simulink model "OFDM_256_pilots"  (R2018b)
settings: Solver=VariableStepAuto  StartTime=0.0  StopTime=inf  RelTol=1e-3
PreLoadFcn:
  | M=16;
  | Fs=1e7;
undefined symbols (not defined in the file): EbNo
libraries: commutil2 x2, commsink2 x2, commofdm x2, commdigbbndam3 x2, commchan3 x1, commrandsrc3 x1
settings Model: Creator=HOBA  LastModifiedBy=HOBA

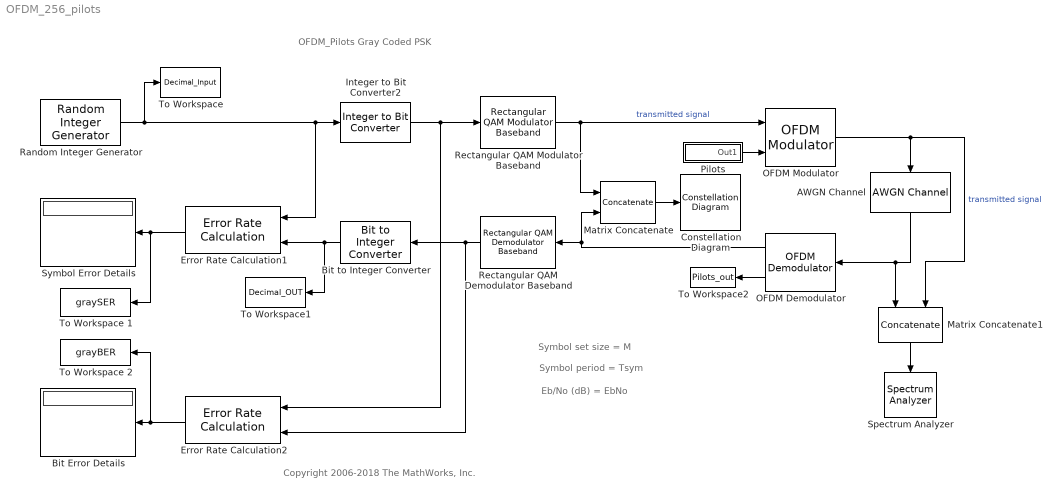
== system OFDM_256_pilots ==
  note: Symbol period = Tsym
  note: Copyright 2006-2018 The MathWorks, Inc.
  note: Symbol set size = M
  note: OFDM_Pilots Gray Coded PSK
  note: Eb/No (dB) = EbNo
  AWGN Channel : commchan3/AWGN Channel  InputProcessing=Columns as channels (frame based)  seed=67  noiseMode="Signal to noise ratio  (Eb/No)"  EbNodB=EbNo  EsNodB=EbNo+10*log10(log2(M))  SNRdB=10  bitsPerSym=320*log2(M)  Ps=1  Tsym=(256/320)*(1/Fs)  variance=1
      settings: SourceProductName=Communications Toolbox
  Bit Error Details : Display
  Bit to Integer Converter : commutil2/Bit to Integer Converter  nbits=log2(M)  bitOrder=MSB first  signedOutputValues=Unsigned  outDtype=Smallest integer  outDtypeSigned=Inherit via internal rule
      settings: SourceProductName=Communications Toolbox
  Constellation Diagram : ConstellationDiagram
  Error Rate Calculation1 : commsink2/Error Rate Calculation  N=0  st_delay=0  cp_mode=Entire frame  subframe=[]  PMode=Port  WsName=SymErrorVec  RsMode2=off  stop=off  numErr=100  maxBits=1e6
      settings: SourceProductName=Communications Toolbox
  Error Rate Calculation2 : commsink2/Error Rate Calculation  N=0  st_delay=0  cp_mode=Entire frame  subframe=[]  PMode=Port  WsName=BitErrorVec  RsMode2=off  stop=on  numErr=1000  maxBits=1e8
      settings: SourceProductName=Communications Toolbox
  Integer to Bit Converter2 : commutil2/Integer to Bit Converter  nbits=log2(M)  signedInputValues=Unsigned  bitOrder=MSB first  outDtype=Smallest unsigned integer
      settings: SourceProductName=Communications Toolbox
  Matrix Concatenate : Concatenate  Mode=Multidimensional array  ConcatenateDimension=2
  Matrix Concatenate1 : Concatenate  Mode=Multidimensional array  ConcatenateDimension=2
  OFDM Demodulator : commofdm/OFDM Demodulator  FFTLength=256  NumGuardBandCarriers=[28; 27]  RemoveDCCarrier=on  PilotOutputPort=on  PilotCarrierIndices=[41; 66; 91; 116; 142; 167; 192; 217]  CyclicPrefixLength=64  NumSymbols=1  NumReceiveAntennas=1  SimulateUsing=Interpreted execution
      settings: SourceProductName=Communications System Toolbox  SourceProductBaseCode=CM
  OFDM Modulator : commofdm/OFDM Modulator  FFTLength=256  NumGuardBandCarriers=[28; 27]  InsertDCNull=on  PilotInputPort=on  PilotCarrierIndices=[41; 66; 91; 116; 142; 167; 192; 217]  CyclicPrefixLength=64  Windowing=off  WindowLength=1  NumSymbols=1  NumTransmitAntennas=1  SimulateUsing=Interpreted execution
      settings: SourceProductName=Communications System Toolbox  SourceProductBaseCode=CM
  Pilots : Subsystem
  Random Integer Generator : commrandsrc3/Random Integer Generator  SetSize=M  SeedSource=Auto  Seed=529558  SampleTime=1/Fs  SamplesPerFrame=192  OutputDataType=uint8  SimulateUsing=Interpreted execution
      settings: SourceProductName=Communications Toolbox
  Rectangular QAM Demodulator Baseband : commdigbbndam3/Rectangular QAM Demodulator Baseband  M=M  OutType=Bit  DecType=Hard decision  VarSource=Dialog  Variance=1  Dec=Gray  Mapping=[0:15]  PowType=Average Power  MinDist=2  AvgPow=1  PeakPow=1  Ph=0  outDtype1=Smallest unsigned integer  outDtype2=Inherit via internal rule  derotateFactorWordLen=16  derotateFactorDataTypeStr=Inherit: Same word length as input  derotateFactorLastDataTypeStr=Inherit: Same word length as input  denormFactorWordLen=16  denormFactorDataTypeStr=Inherit: Same word length as input  denormFactorLastDataTypeStr=Inherit: Same word length as input  prodOutWordLen=32  prodOutOverflowMode=Wrap  prodOutRoundingMode=Floor  prodOutOvFlMode=off  prodOutOvFlModeLastStrValue=off  sumWordLen=32
  Rectangular QAM Modulator Baseband : commdigbbndam3/Rectangular QAM Modulator Baseband  M=M  InType=Bit  Enc=Gray  Mapping=[0:15]  PowType=Average Power  MinDist=2  AvgPow=1  PeakPow=1  Ph=0  outDtype=double  outWordLen=16  outUDDataType=sfix(16)  outFracLenMode=Best precision  outFracLen=15  outDataTypeStr=double  outLastDataTypeStr=double
  Spectrum Analyzer : SpectrumAnalyzer
  Symbol Error Details : Display
  To Workspace : ToWorkspace  VariableName=Decimal_Input  SampleTime=-1
      settings: Save2DSignal=2-D array (concatenate along first dimension)
  To Workspace 1 : ToWorkspace  VariableName=graySER  SampleTime=-1
      settings: MaxDataPoints=1
  To Workspace 2 : ToWorkspace  VariableName=grayBER  SampleTime=-1
      settings: MaxDataPoints=1
  To Workspace1 : ToWorkspace  VariableName=Decimal_OUT  SampleTime=-1
      settings: Save2DSignal=2-D array (concatenate along first dimension)
  To Workspace2 : ToWorkspace  VariableName=Pilots_out  SampleTime=-1
      settings: Save2DSignal=2-D array (concatenate along first dimension)
  wires:
  Rectangular QAM Modulator Baseband/1 -> OFDM Modulator/1, Matrix Concatenate/1  "transmitted signal"
  Integer to Bit Converter2/1 -> Rectangular QAM Modulator Baseband/1, Error Rate Calculation2/1
  Matrix Concatenate1/1 -> Spectrum Analyzer/1
  Bit to Integer Converter/1 -> To Workspace1/1, Error Rate Calculation1/2
  AWGN Channel/1 -> Matrix Concatenate1/1, OFDM Demodulator/1
  Matrix Concatenate/1 -> Constellation Diagram/1
  OFDM Modulator/1 -> Matrix Concatenate1/2, AWGN Channel/1  "transmitted signal"
  Random Integer Generator/1 -> To Workspace/1, Integer to Bit Converter2/1, Error Rate Calculation1/1
  Rectangular QAM Demodulator Baseband/1 -> Bit to Integer Converter/1, Error Rate Calculation2/2
  OFDM Demodulator/1 -> Rectangular QAM Demodulator Baseband/1, Matrix Concatenate/2
  Error Rate Calculation2/1 -> Bit Error Details/1, To Workspace 2/1
  Error Rate Calculation1/1 -> Symbol Error Details/1, To Workspace 1/1
  OFDM Demodulator/2 -> To Workspace2/1
  Pilots/1(Out1) -> OFDM Modulator/2

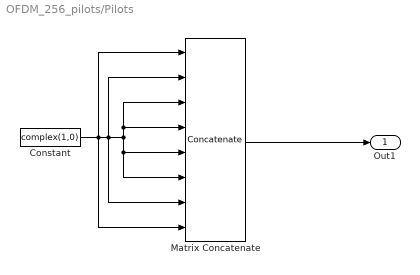
== system OFDM_256_pilots/Pilots ==
  Constant : Constant  Value=complex(1,0)  VectorParams1D=off
  Matrix Concatenate : Concatenate  NumInputs=8  ConcatenateDimension=2
  Out1 : Outport
  wires:
  Constant/1 -> Matrix Concatenate/8, Matrix Concatenate/7, Matrix Concatenate/6, Matrix Concatenate/5, Matrix Concatenate/4, Matrix Concatenate/3, Matrix Concatenate/2, Matrix Concatenate/1
  Matrix Concatenate/1 -> Out1/1
